simulink model "Microgrid_PV_WG_Bat_EV_j_22b"  (R2022b)
settings: Solver=VariableStepAuto  StartTime=0.0  StopTime=1  RelTol=1e-3
undefined symbols (not defined in the file or in its folder): Acid, Ion, Lead, Lithium
libraries: slpidlib x35, spsabctodq0Lib x23, spsSeriesRLCBranchLib x19, spsCurrentMeasurementLib x13, spsVoltageMeasurementLib x11, spsThreePhaseVIMeasurementLib x10, spsPLL3phLib x9, spsThreePhaseSeriesRLCBranchLib x9, spsPower3phInstantaneousLib x8, spsIGBTDiodeLib x8, spsUniversalBridgeLib x7, spsPWMGeneratorDCDCLib x6
(part 2 of 5)

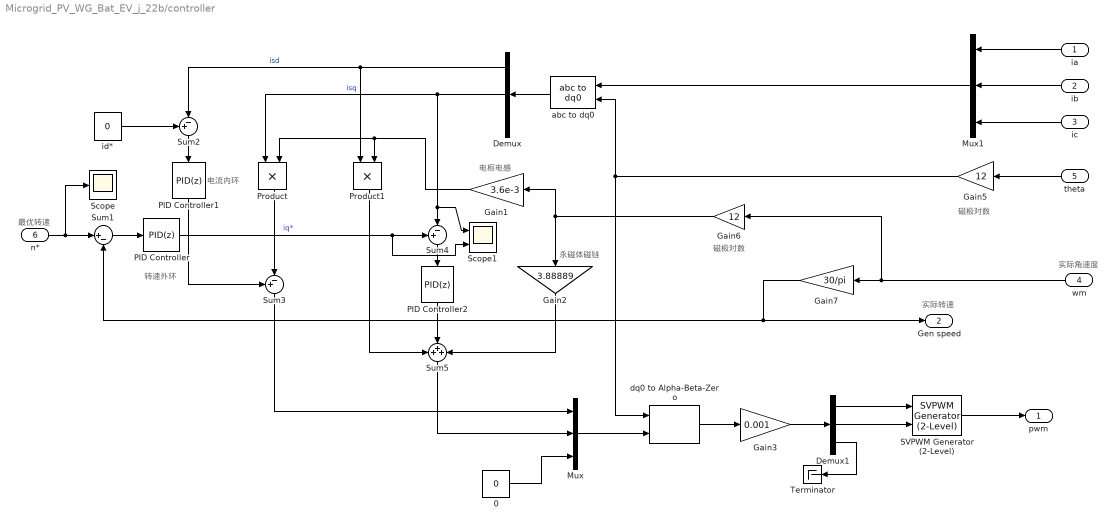
== system Microgrid_PV_WG_Bat_EV_j_22b/controller ==
  note: 电枢电感
  note: 永磁体磁链
  note: 实际角速度
  note: 实际转速
  note: 最优转速
  note: 电流内环
  note: 转速外环
  note: 磁极对数
  note: 磁极对数
  ia : Inport
  ib : Inport  Port=2
  ic : Inport  Port=3
  wm : Inport  Port=4
  theta : Inport  Port=5
  n* : Inport  Port=6
  0 : Constant  Value=0
  Demux : Demux  Outputs=3
  Demux1 : Demux  Outputs=3
  Gain1 : Gain  Gain=3.6e-3
  Gain2 : Gain  Gain=3.88889
  Gain3 : Gain  Gain=0.001
  Gain5 : Gain  Gain=12
  Gain6 : Gain  Gain=12
  Gain7 : Gain  Gain=30/pi
  Mux : Mux  Inputs=3
  Mux1 : Mux  Inputs=3
  PID Controller : slpidlib/PID Controller  Controller=PID  Form=Parallel  TimeDomain=Discrete-time  UseExternalTs=off  SampleTime=1e-5  IntegratorMethod=Forward Euler  FilterMethod=Forward Euler  ControllerParametersSource=internal  P=20  I=400  UseKiTs=off  D=0  N=100  UseFilter=on  TunerSelectOption=Transfer Function Based (PID Tuner App)  InitialConditionSource=internal  InitialConditionForIntegrator=0  InitialConditionForFilter=0  DifferentiatorICPrevScaledInput=0  ExternalReset=none  TrackingMode=off  Kt=1  LimitOutput=off  SatLimitsSource=internal  UpperSaturationLimit=inf  LowerSaturationLimit=-inf  LinearizeAsGain=on  AntiWindupMode=none  Kb=1  LimitIntegrator=off  UpperIntegratorSaturationLimit=inf  LowerIntegratorSaturationLimit=-inf  POutMin=[]  POutMax=[]  IOutMin=[]  IOutMax=[]  DOutMin=[]  DOutMax=[]  NOutMin=[]  NOutMax=[]  SumOutMin=[]  SumOutMax=[]  SaturationOutMin=[]  SaturationOutMax=[]  PParamMin=[]  PParamMax=[]  IParamMin=[]  IParamMax=[]  DParamMin=[]  DParamMax=[]  NParamMin=[]  NParamMax=[]  KbParamMin=[]  KbParamMax=[]  KtParamMin=[]  KtParamMax=[]  KbOutMin=[]  KbOutMax=[]  KtOutMin=[]  KtOutMax=[]  IntegratorOutMin=[]  IntegratorOutMax=[]  FilterOutMin=[]  FilterOutMax=[]  SumI1OutMin=[]  SumI1OutMax=[]  SumI2OutMin=[]  SumI2OutMax=[]  SumI3OutMin=[]  SumI3OutMax=[]  SumI4OutMin=[]  SumI4OutMax=[]  SumDOutMin=[]  SumDOutMax=[]  DifferentiatorOutMin=[]  DifferentiatorOutMax=[]  FilterDiffOutCoefMin=[]  FilterDiffOutCoefMax=[]  ReciprocalOutMin=[]  ReciprocalOutMax=[]  SumDenOutMin=[]  SumDenOutMax=[]  SumNumOutMin=[]  SumNumOutMax=[]  DivideOutMin=[]  DivideOutMax=[]  UdiffTsProdOutMin=[]  UdiffTsProdOutMax=[]  NTsProdOutMin=[]  NTsProdOutMax=[]  UintegralTsProdOutMin=[]  UintegralTsProdOutMax=[]  UngainTsProdOutMin=[]  UngainTsProdOutMax=[]  IntegratorContinuousStateAttributes=''  IntegratorStateMustResolveToSignalObject=off  IntegratorRTWStateStorageClass=Auto  FilterContinuousStateAttributes=''  FilterStateMustResolveToSignalObject=off  FilterRTWStateStorageClass=Auto  ParallelPVariant=InternalParameters  IdealPVariant=Disabled  IVariant=InternalParameters  DVariant=InternalParameters  IntegratorVariant=Discrete  SatVariant=Disabled  AWVariant=Passthrough  PCopyVariant=Disabled  TRVariant=Disabled  FdbkBlocksVariant=Forward  IdealPFdbkVariant=Disabled  SatFdbkVariant=Disabled  DerivativeFilterVariant=ForwardEulerFilter  NVariant=InternalParameters  NCopyVariant=Disabled  FilterICVariant=InternalICsFilter  IntegratorICVariant=InternalICs  ExternalResetVariant=Disabled  TRSumVariant=Passthrough  SumFdbkVariant=Disabled  SumVariant=Sum_PID  TsampFilterVariant=InternalTs  TsampNgainVariant=Passthrough  TsampIntegralVariant=Disabled_SignalSpec  ExternalSaturationOutDataTypeStr=Inherit: Same as second input
  PID Controller1 : slpidlib/PID Controller  Controller=PID  Form=Parallel  TimeDomain=Discrete-time  UseExternalTs=off  SampleTime=1e-5  IntegratorMethod=Forward Euler  FilterMethod=Forward Euler  ControllerParametersSource=internal  P=5  I=100  UseKiTs=off  D=0  N=100  UseFilter=on  TunerSelectOption=Transfer Function Based (PID Tuner App)  InitialConditionSource=internal  InitialConditionForIntegrator=0  InitialConditionForFilter=0  DifferentiatorICPrevScaledInput=0  ExternalReset=none  TrackingMode=off  Kt=1  LimitOutput=off  SatLimitsSource=internal  UpperSaturationLimit=inf  LowerSaturationLimit=-inf  LinearizeAsGain=on  AntiWindupMode=none  Kb=1  LimitIntegrator=off  UpperIntegratorSaturationLimit=inf  LowerIntegratorSaturationLimit=-inf  POutMin=[]  POutMax=[]  IOutMin=[]  IOutMax=[]  DOutMin=[]  DOutMax=[]  NOutMin=[]  NOutMax=[]  SumOutMin=[]  SumOutMax=[]  SaturationOutMin=[]  SaturationOutMax=[]  PParamMin=[]  PParamMax=[]  IParamMin=[]  IParamMax=[]  DParamMin=[]  DParamMax=[]  NParamMin=[]  NParamMax=[]  KbParamMin=[]  KbParamMax=[]  KtParamMin=[]  KtParamMax=[]  KbOutMin=[]  KbOutMax=[]  KtOutMin=[]  KtOutMax=[]  IntegratorOutMin=[]  IntegratorOutMax=[]  FilterOutMin=[]  FilterOutMax=[]  SumI1OutMin=[]  SumI1OutMax=[]  SumI2OutMin=[]  SumI2OutMax=[]  SumI3OutMin=[]  SumI3OutMax=[]  SumI4OutMin=[]  SumI4OutMax=[]  SumDOutMin=[]  SumDOutMax=[]  DifferentiatorOutMin=[]  DifferentiatorOutMax=[]  FilterDiffOutCoefMin=[]  FilterDiffOutCoefMax=[]  ReciprocalOutMin=[]  ReciprocalOutMax=[]  SumDenOutMin=[]  SumDenOutMax=[]  SumNumOutMin=[]  SumNumOutMax=[]  DivideOutMin=[]  DivideOutMax=[]  UdiffTsProdOutMin=[]  UdiffTsProdOutMax=[]  NTsProdOutMin=[]  NTsProdOutMax=[]  UintegralTsProdOutMin=[]  UintegralTsProdOutMax=[]  UngainTsProdOutMin=[]  UngainTsProdOutMax=[]  IntegratorContinuousStateAttributes=''  IntegratorStateMustResolveToSignalObject=off  IntegratorRTWStateStorageClass=Auto  FilterContinuousStateAttributes=''  FilterStateMustResolveToSignalObject=off  FilterRTWStateStorageClass=Auto  ParallelPVariant=InternalParameters  IdealPVariant=Disabled  IVariant=InternalParameters  DVariant=InternalParameters  IntegratorVariant=Discrete  SatVariant=Disabled  AWVariant=Passthrough  PCopyVariant=Disabled  TRVariant=Disabled  FdbkBlocksVariant=Forward  IdealPFdbkVariant=Disabled  SatFdbkVariant=Disabled  DerivativeFilterVariant=ForwardEulerFilter  NVariant=InternalParameters  NCopyVariant=Disabled  FilterICVariant=InternalICsFilter  IntegratorICVariant=InternalICs  ExternalResetVariant=Disabled  TRSumVariant=Passthrough  SumFdbkVariant=Disabled  SumVariant=Sum_PID  TsampFilterVariant=InternalTs  TsampNgainVariant=Passthrough  TsampIntegralVariant=Disabled_SignalSpec  ExternalSaturationOutDataTypeStr=Inherit: Same as second input
  PID Controller2 : slpidlib/PID Controller  Controller=PID  Form=Parallel  TimeDomain=Discrete-time  UseExternalTs=off  SampleTime=1e-5  IntegratorMethod=Forward Euler  FilterMethod=Forward Euler  ControllerParametersSource=internal  P=5  I=100  UseKiTs=off  D=0  N=100  UseFilter=on  TunerSelectOption=Transfer Function Based (PID Tuner App)  InitialConditionSource=internal  InitialConditionForIntegrator=0  InitialConditionForFilter=0  DifferentiatorICPrevScaledInput=0  ExternalReset=none  TrackingMode=off  Kt=1  LimitOutput=off  SatLimitsSource=internal  UpperSaturationLimit=inf  LowerSaturationLimit=-inf  LinearizeAsGain=on  AntiWindupMode=none  Kb=1  LimitIntegrator=off  UpperIntegratorSaturationLimit=inf  LowerIntegratorSaturationLimit=-inf  POutMin=[]  POutMax=[]  IOutMin=[]  IOutMax=[]  DOutMin=[]  DOutMax=[]  NOutMin=[]  NOutMax=[]  SumOutMin=[]  SumOutMax=[]  SaturationOutMin=[]  SaturationOutMax=[]  PParamMin=[]  PParamMax=[]  IParamMin=[]  IParamMax=[]  DParamMin=[]  DParamMax=[]  NParamMin=[]  NParamMax=[]  KbParamMin=[]  KbParamMax=[]  KtParamMin=[]  KtParamMax=[]  KbOutMin=[]  KbOutMax=[]  KtOutMin=[]  KtOutMax=[]  IntegratorOutMin=[]  IntegratorOutMax=[]  FilterOutMin=[]  FilterOutMax=[]  SumI1OutMin=[]  SumI1OutMax=[]  SumI2OutMin=[]  SumI2OutMax=[]  SumI3OutMin=[]  SumI3OutMax=[]  SumI4OutMin=[]  SumI4OutMax=[]  SumDOutMin=[]  SumDOutMax=[]  DifferentiatorOutMin=[]  DifferentiatorOutMax=[]  FilterDiffOutCoefMin=[]  FilterDiffOutCoefMax=[]  ReciprocalOutMin=[]  ReciprocalOutMax=[]  SumDenOutMin=[]  SumDenOutMax=[]  SumNumOutMin=[]  SumNumOutMax=[]  DivideOutMin=[]  DivideOutMax=[]  UdiffTsProdOutMin=[]  UdiffTsProdOutMax=[]  NTsProdOutMin=[]  NTsProdOutMax=[]  UintegralTsProdOutMin=[]  UintegralTsProdOutMax=[]  UngainTsProdOutMin=[]  UngainTsProdOutMax=[]  IntegratorContinuousStateAttributes=''  IntegratorStateMustResolveToSignalObject=off  IntegratorRTWStateStorageClass=Auto  FilterContinuousStateAttributes=''  FilterStateMustResolveToSignalObject=off  FilterRTWStateStorageClass=Auto  ParallelPVariant=InternalParameters  IdealPVariant=Disabled  IVariant=InternalParameters  DVariant=InternalParameters  IntegratorVariant=Discrete  SatVariant=Disabled  AWVariant=Passthrough  PCopyVariant=Disabled  TRVariant=Disabled  FdbkBlocksVariant=Forward  IdealPFdbkVariant=Disabled  SatFdbkVariant=Disabled  DerivativeFilterVariant=ForwardEulerFilter  NVariant=InternalParameters  NCopyVariant=Disabled  FilterICVariant=InternalICsFilter  IntegratorICVariant=InternalICs  ExternalResetVariant=Disabled  TRSumVariant=Passthrough  SumFdbkVariant=Disabled  SumVariant=Sum_PID  TsampFilterVariant=InternalTs  TsampNgainVariant=Passthrough  TsampIntegralVariant=Disabled_SignalSpec  ExternalSaturationOutDataTypeStr=Inherit: Same as second input
  Product : Product
  Product1 : Product
  SVPWM Generator (2-Level) : spsSVPWMGenerator2LevelLib/SVPWM Generator (2-Level)  InputType=alpha-beta components  SwitchingPattern=Pattern #1  Fc=3000  ParUref=[0.8 -30 50]  Ts=0
  Scope : Scope
  Scope1 : Scope  NumInputPorts=2
  Sum1 : Sum  Inputs=|+-
  Sum2 : Sum  Inputs=+-|
  Sum3 : Sum  Inputs=+-|
  Sum4 : Sum  Inputs=+-|
  Sum5 : Sum  Inputs=+++
  Terminator : Terminator
  abc to dq0 : spsabctodq0Lib/abc to dq0  Alignment=90 degrees behind phase A axis
  dq0 to Alpha-Beta-Zero : spsdq0toAlphaBetaZeroLib/dq0 to Alpha-Beta-Zero  Alignment=90 degrees behind phase A axis
  id* : Constant  Value=0
  pwm : Outport
  Gen speed : Outport  Port=2
  wires:
  Demux1/1 -> SVPWM Generator (2-Level)/1
  Gain5/1 -> dq0 to Alpha-Beta-Zero/2, abc to dq0/2
  Gain7/1 -> Gen speed/1, Sum1/2
  Mux/1 -> dq0 to Alpha-Beta-Zero/1
  wm/1 -> Gain6/1, Gain7/1
  Mux1/1 -> abc to dq0/1
  ib/1 -> Mux1/2
  Sum3/1 -> Mux/1
  PID Controller2/1 -> Sum5/2
  Sum1/1 -> PID Controller/1
  0/1 -> Mux/3
  Gain6/1 -> Gain1/1, Gain2/1
  theta/1 -> Gain5/1
  Demux/2 -> Scope1/1, Sum4/2, Product/1  "isq"
  Demux1/3 -> Terminator/1
  Gain3/1 -> Demux1/1
  dq0 to Alpha-Beta-Zero/1 -> Gain3/1
  Sum5/1 -> Mux/2
  Demux/1 -> Sum2/2, Product1/1  "isd"
  id*/1 -> Sum2/1
  Gain1/1 -> Product1/2, Product/2
  ia/1 -> Mux1/1
  PID Controller1/1 -> Sum3/1
  SVPWM Generator (2-Level)/1 -> pwm/1
  Product1/1 -> Sum5/1
  Demux1/2 -> SVPWM Generator (2-Level)/2
  Product/1 -> Sum3/2
  PID Controller/1 -> Scope1/2, Sum4/1  "iq*"
  Sum2/1 -> PID Controller1/1
  Gain2/1 -> Sum5/3
  Sum4/1 -> PID Controller2/1
  ic/1 -> Mux1/3
  abc to dq0/1 -> Demux/1
  n*/1 -> Scope/1, Sum1/1

== system Microgrid_PV_WG_Bat_EV_j_22b/controller2 ==
  note: abc2dq
  Udc : Inport
  Udc_ref : Inport  Port=2
  Vabc : Inport  Port=3
  Iabc : Inport  Port=4
  Constant : Constant  Commented=on  Value=600
  Constant4 : Constant  Value=0
  Demux2 : Demux  Outputs=3
  Demux3 : Demux  Outputs=3
  Demux4 : Demux  Outputs=3
  Gain6 : Gain  Gain=2*pi*50*(7e-3)
  Gain7 : Gain  Gain=2*pi*50*(7e-3)
  Gain9 : Gain  Gain=0.001
  Mux1 : Mux  Inputs=3
  PID 3 : slpidlib/PID Controller  Controller=PID  Form=Parallel  TimeDomain=Discrete-time  UseExternalTs=off  SampleTime=1e-5  IntegratorMethod=Forward Euler  FilterMethod=Forward Euler  ControllerParametersSource=internal  P=2  I=70  UseKiTs=off  D=0  N=100  UseFilter=on  TunerSelectOption=Transfer Function Based (PID Tuner App)  InitialConditionSource=internal  InitialConditionForIntegrator=0  InitialConditionForFilter=0  DifferentiatorICPrevScaledInput=0  ExternalReset=none  TrackingMode=off  Kt=1  LimitOutput=off  SatLimitsSource=internal  UpperSaturationLimit=inf  LowerSaturationLimit=-inf  LinearizeAsGain=on  AntiWindupMode=none  Kb=1  LimitIntegrator=off  UpperIntegratorSaturationLimit=inf  LowerIntegratorSaturationLimit=-inf  POutMin=[]  POutMax=[]  IOutMin=[]  IOutMax=[]  DOutMin=[]  DOutMax=[]  NOutMin=[]  NOutMax=[]  SumOutMin=[]  SumOutMax=[]  SaturationOutMin=[]  SaturationOutMax=[]  PParamMin=[]  PParamMax=[]  IParamMin=[]  IParamMax=[]  DParamMin=[]  DParamMax=[]  NParamMin=[]  NParamMax=[]  KbParamMin=[]  KbParamMax=[]  KtParamMin=[]  KtParamMax=[]  KbOutMin=[]  KbOutMax=[]  KtOutMin=[]  KtOutMax=[]  IntegratorOutMin=[]  IntegratorOutMax=[]  FilterOutMin=[]  FilterOutMax=[]  SumI1OutMin=[]  SumI1OutMax=[]  SumI2OutMin=[]  SumI2OutMax=[]  SumI3OutMin=[]  SumI3OutMax=[]  SumI4OutMin=[]  SumI4OutMax=[]  SumDOutMin=[]  SumDOutMax=[]  DifferentiatorOutMin=[]  DifferentiatorOutMax=[]  FilterDiffOutCoefMin=[]  FilterDiffOutCoefMax=[]  ReciprocalOutMin=[]  ReciprocalOutMax=[]  SumDenOutMin=[]  SumDenOutMax=[]  SumNumOutMin=[]  SumNumOutMax=[]  DivideOutMin=[]  DivideOutMax=[]  UdiffTsProdOutMin=[]  UdiffTsProdOutMax=[]  NTsProdOutMin=[]  NTsProdOutMax=[]  UintegralTsProdOutMin=[]  UintegralTsProdOutMax=[]  UngainTsProdOutMin=[]  UngainTsProdOutMax=[]  IntegratorContinuousStateAttributes=''  IntegratorStateMustResolveToSignalObject=off  IntegratorRTWStateStorageClass=Auto  FilterContinuousStateAttributes=''  FilterStateMustResolveToSignalObject=off  FilterRTWStateStorageClass=Auto  ParallelPVariant=InternalParameters  IdealPVariant=Disabled  IVariant=InternalParameters  DVariant=InternalParameters  IntegratorVariant=Discrete  SatVariant=Disabled  AWVariant=Passthrough  PCopyVariant=Disabled  TRVariant=Disabled  FdbkBlocksVariant=Forward  IdealPFdbkVariant=Disabled  SatFdbkVariant=Disabled  DerivativeFilterVariant=ForwardEulerFilter  NVariant=InternalParameters  NCopyVariant=Disabled  FilterICVariant=InternalICsFilter  IntegratorICVariant=InternalICs  ExternalResetVariant=Disabled  TRSumVariant=Passthrough  SumFdbkVariant=Disabled  SumVariant=Sum_PID  TsampFilterVariant=InternalTs  TsampNgainVariant=Passthrough  TsampIntegralVariant=Disabled_SignalSpec  ExternalSaturationOutDataTypeStr=Inherit: Same as second input
  PID 4 : slpidlib/PID Controller  Controller=PID  Form=Parallel  TimeDomain=Discrete-time  UseExternalTs=off  SampleTime=1e-5  IntegratorMethod=Forward Euler  FilterMethod=Forward Euler  ControllerParametersSource=internal  P=1  I=15  UseKiTs=off  D=0  N=100  UseFilter=on  TunerSelectOption=Transfer Function Based (PID Tuner App)  InitialConditionSource=internal  InitialConditionForIntegrator=0  InitialConditionForFilter=0  DifferentiatorICPrevScaledInput=0  ExternalReset=none  TrackingMode=off  Kt=1  LimitOutput=off  SatLimitsSource=internal  UpperSaturationLimit=inf  LowerSaturationLimit=-inf  LinearizeAsGain=on  AntiWindupMode=none  Kb=1  LimitIntegrator=off  UpperIntegratorSaturationLimit=inf  LowerIntegratorSaturationLimit=-inf  POutMin=[]  POutMax=[]  IOutMin=[]  IOutMax=[]  DOutMin=[]  DOutMax=[]  NOutMin=[]  NOutMax=[]  SumOutMin=[]  SumOutMax=[]  SaturationOutMin=[]  SaturationOutMax=[]  PParamMin=[]  PParamMax=[]  IParamMin=[]  IParamMax=[]  DParamMin=[]  DParamMax=[]  NParamMin=[]  NParamMax=[]  KbParamMin=[]  KbParamMax=[]  KtParamMin=[]  KtParamMax=[]  KbOutMin=[]  KbOutMax=[]  KtOutMin=[]  KtOutMax=[]  IntegratorOutMin=[]  IntegratorOutMax=[]  FilterOutMin=[]  FilterOutMax=[]  SumI1OutMin=[]  SumI1OutMax=[]  SumI2OutMin=[]  SumI2OutMax=[]  SumI3OutMin=[]  SumI3OutMax=[]  SumI4OutMin=[]  SumI4OutMax=[]  SumDOutMin=[]  SumDOutMax=[]  DifferentiatorOutMin=[]  DifferentiatorOutMax=[]  FilterDiffOutCoefMin=[]  FilterDiffOutCoefMax=[]  ReciprocalOutMin=[]  ReciprocalOutMax=[]  SumDenOutMin=[]  SumDenOutMax=[]  SumNumOutMin=[]  SumNumOutMax=[]  DivideOutMin=[]  DivideOutMax=[]  UdiffTsProdOutMin=[]  UdiffTsProdOutMax=[]  NTsProdOutMin=[]  NTsProdOutMax=[]  UintegralTsProdOutMin=[]  UintegralTsProdOutMax=[]  UngainTsProdOutMin=[]  UngainTsProdOutMax=[]  IntegratorContinuousStateAttributes=''  IntegratorStateMustResolveToSignalObject=off  IntegratorRTWStateStorageClass=Auto  FilterContinuousStateAttributes=''  FilterStateMustResolveToSignalObject=off  FilterRTWStateStorageClass=Auto  ParallelPVariant=InternalParameters  IdealPVariant=Disabled  IVariant=InternalParameters  DVariant=InternalParameters  IntegratorVariant=Discrete  SatVariant=Disabled  AWVariant=Passthrough  PCopyVariant=Disabled  TRVariant=Disabled  FdbkBlocksVariant=Forward  IdealPFdbkVariant=Disabled  SatFdbkVariant=Disabled  DerivativeFilterVariant=ForwardEulerFilter  NVariant=InternalParameters  NCopyVariant=Disabled  FilterICVariant=InternalICsFilter  IntegratorICVariant=InternalICs  ExternalResetVariant=Disabled  TRSumVariant=Passthrough  SumFdbkVariant=Disabled  SumVariant=Sum_PID  TsampFilterVariant=InternalTs  TsampNgainVariant=Passthrough  TsampIntegralVariant=Disabled_SignalSpec  ExternalSaturationOutDataTypeStr=Inherit: Same as second input
  PID 5 : slpidlib/PID Controller  Controller=PID  Form=Parallel  TimeDomain=Discrete-time  UseExternalTs=off  SampleTime=1e-5  IntegratorMethod=Forward Euler  FilterMethod=Forward Euler  ControllerParametersSource=internal  P=1  I=15  UseKiTs=off  D=0  N=100  UseFilter=on  TunerSelectOption=Transfer Function Based (PID Tuner App)  InitialConditionSource=internal  InitialConditionForIntegrator=0  InitialConditionForFilter=0  DifferentiatorICPrevScaledInput=0  ExternalReset=none  TrackingMode=off  Kt=1  LimitOutput=off  SatLimitsSource=internal  UpperSaturationLimit=inf  LowerSaturationLimit=-inf  LinearizeAsGain=on  AntiWindupMode=none  Kb=1  LimitIntegrator=off  UpperIntegratorSaturationLimit=inf  LowerIntegratorSaturationLimit=-inf  POutMin=[]  POutMax=[]  IOutMin=[]  IOutMax=[]  DOutMin=[]  DOutMax=[]  NOutMin=[]  NOutMax=[]  SumOutMin=[]  SumOutMax=[]  SaturationOutMin=[]  SaturationOutMax=[]  PParamMin=[]  PParamMax=[]  IParamMin=[]  IParamMax=[]  DParamMin=[]  DParamMax=[]  NParamMin=[]  NParamMax=[]  KbParamMin=[]  KbParamMax=[]  KtParamMin=[]  KtParamMax=[]  KbOutMin=[]  KbOutMax=[]  KtOutMin=[]  KtOutMax=[]  IntegratorOutMin=[]  IntegratorOutMax=[]  FilterOutMin=[]  FilterOutMax=[]  SumI1OutMin=[]  SumI1OutMax=[]  SumI2OutMin=[]  SumI2OutMax=[]  SumI3OutMin=[]  SumI3OutMax=[]  SumI4OutMin=[]  SumI4OutMax=[]  SumDOutMin=[]  SumDOutMax=[]  DifferentiatorOutMin=[]  DifferentiatorOutMax=[]  FilterDiffOutCoefMin=[]  FilterDiffOutCoefMax=[]  ReciprocalOutMin=[]  ReciprocalOutMax=[]  SumDenOutMin=[]  SumDenOutMax=[]  SumNumOutMin=[]  SumNumOutMax=[]  DivideOutMin=[]  DivideOutMax=[]  UdiffTsProdOutMin=[]  UdiffTsProdOutMax=[]  NTsProdOutMin=[]  NTsProdOutMax=[]  UintegralTsProdOutMin=[]  UintegralTsProdOutMax=[]  UngainTsProdOutMin=[]  UngainTsProdOutMax=[]  IntegratorContinuousStateAttributes=''  IntegratorStateMustResolveToSignalObject=off  IntegratorRTWStateStorageClass=Auto  FilterContinuousStateAttributes=''  FilterStateMustResolveToSignalObject=off  FilterRTWStateStorageClass=Auto  ParallelPVariant=InternalParameters  IdealPVariant=Disabled  IVariant=InternalParameters  DVariant=InternalParameters  IntegratorVariant=Discrete  SatVariant=Disabled  AWVariant=Passthrough  PCopyVariant=Disabled  TRVariant=Disabled  FdbkBlocksVariant=Forward  IdealPFdbkVariant=Disabled  SatFdbkVariant=Disabled  DerivativeFilterVariant=ForwardEulerFilter  NVariant=InternalParameters  NCopyVariant=Disabled  FilterICVariant=InternalICsFilter  IntegratorICVariant=InternalICs  ExternalResetVariant=Disabled  TRSumVariant=Passthrough  SumFdbkVariant=Disabled  SumVariant=Sum_PID  TsampFilterVariant=InternalTs  TsampNgainVariant=Passthrough  TsampIntegralVariant=Disabled_SignalSpec  ExternalSaturationOutDataTypeStr=Inherit: Same as second input
  PLL (3ph)1 : spsPLL3phLib/PLL (3ph)  Fmin=45  Par_Init=[0, 50]  ParK=[180, 3200, 1]  TcD=1e-4  MaxRateChangeFreq=12  FilterCutOffFreq=25  Ts=0  AGC=on
  SVPWM Generator (2-Level)1 : spsSVPWMGenerator2LevelLib/SVPWM Generator (2-Level)  InputType=alpha-beta components  SwitchingPattern=Pattern #1  Fc=10000  ParUref=[0.8 -30 50]  Ts=0
  Sum1 : Sum  Commented=on  Inputs=|+-
  Sum5 : Sum  Inputs=|+-
  Sum6 : Sum  Inputs=|+-
  Sum7 : Sum  Inputs=++-
  Sum8 : Sum  Inputs=-+|
  Sum9 : Sum  Inputs=+++
  Terminator2 : Terminator
  Terminator3 : Terminator
  Terminator4 : Terminator
  abc to dq1 : spsabctodq0Lib/abc to dq0  Alignment=90 degrees behind phase A axis
  abc to dq2 : spsabctodq0Lib/abc to dq0  Alignment=90 degrees behind phase A axis
  dq0 to Alpha-Beta-Zero1 : spsdq0toAlphaBetaZeroLib/dq0 to Alpha-Beta-Zero  Alignment=90 degrees behind phase A axis
  iq*=0 : Constant  Value=0
  Pulse : Outport
  wires:
  Sum5/1 -> PID 3/1  "d"
  Gain6/1 -> Sum7/3
  Demux2/1 -> Sum7/1  "Vd"
  PID 3/1 -> Sum6/1  "id*"
  dq0 to Alpha-Beta-Zero1/1 -> Gain9/1
  PLL (3ph)1/2 -> dq0 to Alpha-Beta-Zero1/2, abc to dq2/2, abc to dq1/2
  Sum6/1 -> PID 4/1
  PID 4/1 -> Sum7/2
  Demux4/3 -> Terminator4/1
  PID 5/1 -> Sum9/2
  Iabc/1 -> abc to dq2/1
  Constant4/1 -> Mux1/3
  Demux3/3 -> Terminator3/1
  abc to dq1/1 -> Demux2/1
  Demux2/3 -> Terminator2/1
  Udc/1 -> Sum5/1
  abc to dq2/1 -> Demux3/1
  iq*=0/1 -> Sum8/2
  SVPWM Generator (2-Level)1/1 -> Pulse/1
  Gain9/1 -> Demux4/1
  Demux3/2 -> Sum8/1, Gain6/1  "iq"
  Demux3/1 -> Gain7/1, Sum6/2  "id"
  Sum7/1 -> Mux1/1  "Ud*"
  Sum8/1 -> PID 5/1
  Sum9/1 -> Mux1/2  "Uq*"
  Mux1/1 -> dq0 to Alpha-Beta-Zero1/1
  Demux4/1 -> SVPWM Generator (2-Level)1/1
  Demux4/2 -> SVPWM Generator (2-Level)1/2
  Udc_ref/1 -> Sum5/2
  Gain7/1 -> Sum9/3
  Demux2/2 -> Sum9/1  "Vq"
  Vabc/1 -> PLL (3ph)1/1, abc to dq1/1  "d"
  Constant/1 -> Sum1/2

== system Microgrid_PV_WG_Bat_EV_j_22b/储氢罐 ==
  Velec : Inport
  L/min : Inport  Port=2
  Add1 : Sum  Inputs=+-
  Add2 : Sum
  Add3 : Sum
  Divide1 : Product  Inputs=*/
  Gain : Gain  Gain=10
  Gain1 : Gain  Gain=30
  Integrator : Integrator
  Product1 : Product  Inputs=***/
  R : Constant  Value=8.3145
  T/C : Constant  Value=25
  conversion : Constant  Value=273.15
  储氢罐的体积/m³ : Constant
  标准大气压/pa : Constant  Value=101325
  标准大气压/pa1 : Constant  Value=101325
  氢气消耗速率转换 : Subsystem
  百分比 : Gain  Gain=100
  SOH : Outport
  wires:
  R/1 -> Product1/2
  Gain/1 -> Add3/2  "储氢罐已有氢气的压强"
  Integrator/1 -> Product1/1
  T/C/1 -> Add2/1
  conversion/1 -> Add2/2
  标准大气压/pa/1 -> Gain/1
  Velec/1 -> Add1/1
  标准大气压/pa1/1 -> Gain1/1
  储氢罐的体积/m³/1 -> Product1/4
  氢气消耗速率转换/1(mol/s) -> Add1/2
  Divide1/1 -> 百分比/1
  Add3/1 -> Divide1/1
  Product1/1 -> Add3/1
  百分比/1 -> SOH/1
  Gain1/1 -> Divide1/2  "储氢罐最大储氢的氢气的压强"
  Add2/1 -> Product1/3  "T/K"
  Add1/1 -> Integrator/1
  L/min/1 -> 氢气消耗速率转换/1(L/min)

== system Microgrid_PV_WG_Bat_EV_j_22b/充电桩 ==
  Battery1 : spsBatteryLib/Battery  BatType=Lead-Acid  ShowTempParam=off  ThermalPreset=no  ShowAgeParam=off  NomV=500  NomQ=1000  SOC=50  Batt_Tr=30  PresetModel=on  MaxQ=1041.6667  MinV=375  FullV=544.4079  Dis_rate=200  R=0.005  Normal_OP=310.2778  expZone="[509.0461      3.333333]"  current=[6.5 13 32.5]  Units=Time  Tci=20  NomT=20  T2=-30  MaxQ2=4.8  FullV2=7.1  Normal_OP2=5.655  expZone2="[6.58           1]"  Rca=0.6  ti=2000  Dp=0  Neq0=0  Tsim=1e6  Ta1=25  Qeol=5.4*0.9  Reol=0.013333*1.2  Char_age=[2.3478, 3]  Dis_age=[2.3478, 10]  N1=1500  N2=10500  N3=1000  N4=1400  Ta2=45  N5=950
  Bus Selector1 : BusSelector  OutputSignals=SOC (%),Current (A),Voltage (V)
  Current Measurement2 : spsCurrentMeasurementLib/Current Measurement  PhasorSimulation=off  OutputType=Complex  PSBequivalent=0
  IGBT/Diode2 : spsIGBTDiodeLib/IGBT//Diode  Ron=1e-3  Rs=1e5  Cs=inf  Measurements=on
  IGBT/Diode3 : spsIGBTDiodeLib/IGBT//Diode  Ron=1e-3  Rs=1e5  Cs=inf  Measurements=on
  Mosfet : spsMosfetLib/Mosfet  Ron=0.1  Lon=0  Rd=0.01  Vfd=0  IC=0  Rs=1e5  Cs=inf  Measurements=on
  PWM Generator (DC-DC)2 : spsPWMGeneratorDCDCLib/PWM Generator (DC-DC)  Fsw=1e4  Ts=0
  Scope : Scope
  Scope3 : Scope  NumInputPorts=2
  Scope5 : Scope  NumInputPorts=3
  Series RLC Branch3 : spsSeriesRLCBranchLib/Series RLC Branch  LConnTagsString=__new0  RConnTagsString=__new0  BranchType=L  Resistance=1  Inductance=11e-2  SetiL0=off  InitialCurrent=0  Capacitance=1e-6  Setx0=off  InitialVoltage=0  Measurements=None
  Series RLC Branch5 : spsSeriesRLCBranchLib/Series RLC Branch  LConnTagsString=__new0  RConnTagsString=__new0  BranchType=RC  Resistance=0.01  Inductance=1e-3  SetiL0=off  InitialCurrent=0  Capacitance=2e-2  Setx0=off  InitialVoltage=10  Measurements=None
  Voltage Measurement1 : spsVoltageMeasurementLib/Voltage Measurement  PhasorSimulation=off  OutputType=Complex  PSBequivalent=0
  恒流恒压充电 : Subsystem
  + : PMIOPort  Side=Right
  - : PMIOPort  Port=2  Side=Right
  Vbat : Outport
  Ibat : Outport  Port=2
  SOC : Outport  Port=3
  wires:
  恒流恒压充电/1(D) -> PWM Generator (DC-DC)2/1, Scope/1
  Bus Selector1/2 -> Scope5/2, [I_Bat]  "<Current (A)>"
  Bus Selector1/1 -> Scope5/1, [SOC]  "<SOC (%)>"
  Voltage Measurement1/1 -> 恒流恒压充电/1(V), Scope3/2
  PWM Generator (DC-DC)2/1 -> Mosfet/1
  Current Measurement2/1 -> Scope3/1, 恒流恒压充电/2(I)
  Battery1/1 -> Bus Selector1/1
  [I_Bat] -> Ibat/1
  Bus Selector1/3 -> Scope5/3, [V_Bat]  "<Voltage (V)>"
  [V_Bat] -> Vbat/1
  [SOC] -> SOC/1
  connections:
  IGBT/Diode2/RConn1 -- Voltage Measurement1/LConn2 -- Battery1/LConn2 -- Series RLC Branch5/RConn1 -- -/RConn1
  Current Measurement2/LConn1 -- Series RLC Branch5/LConn1 -- Series RLC Branch3/RConn1
  +/RConn1 -- Mosfet/LConn1
  IGBT/Diode3/RConn1 -- Current Measurement2/RConn1
  Voltage Measurement1/LConn1 -- IGBT/Diode3/LConn1 -- Battery1/LConn1
  Mosfet/RConn1 -- IGBT/Diode2/LConn1 -- Series RLC Branch3/LConn1

== system Microgrid_PV_WG_Bat_EV_j_22b/光伏 ==
  PV_change : Inport
  Bus Selector : BusSelector  OutputSignals=V_PV,I_PV
  Constant : Constant  Value=25
  Constant1 : Constant  Value=1000
  Constant2 : Constant  Value=1000
  Current Measurement : spsCurrentMeasurementLib/Current Measurement  PhasorSimulation=off  OutputType=Complex  PSBequivalent=0
  Diode : spsDiodeLib/Diode  Ron=0.001  Lon=0  Vf=0.8  IC=0  UseSnubber=0  Rs=500  Cs=250e-9  Measurements=on
  IGBT : spsIGBTLib/IGBT  Ron=0.001  Lon=0  Vf=1  Tf=1e-6  Tt=2e-6  IC=0  Rs=1e5  Cs=inf  Measurements=on
  "PV Array " : spsPVArrayLib/PV Array  Npar=5  Nser=14  PlotType=array @ 25 deg.C & specified irradiances  S_vec="[ 1000  600  100 ]"  Temp_C_vec="[ 45 25  ]"  ModuleName=User-defined  PlotWhenSelected=off  Pm=213.15  Ncell=60  Voc=36.3  Isc=7.84  Vm=29  Im=7.35  beta_Voc_pc=-0.36099  alpha_Isc_pc=0.102  beta_Voc=-0.13104  alpha_Isc=0.0079968  IL=7.8654  I0=2.9273e-10  nI=0.98119  Rsh=313.0553  Rs=0.39381  RobustModel=off  RobustCellTemperature=313.3991  BAL=on  Tc=1e-6  Tfilter=5e-5
  PWM Generator (DC-DC) : spsPWMGeneratorDCDCLib/PWM Generator (DC-DC)  Fsw=15e3  Ts=0
  Scope : Scope
  Series RLC Branch : spsSeriesRLCBranchLib/Series RLC Branch  LConnTagsString=__new0  RConnTagsString=__new0  BranchType=C  Resistance=0.1  Inductance=1e-3  SetiL0=off  InitialCurrent=0  Capacitance=1e-4  Setx0=on  InitialVoltage=400  Measurements=None
  Series RLC Branch1 : spsSeriesRLCBranchLib/Series RLC Branch  LConnTagsString=__new0  RConnTagsString=__new0  BranchType=L  Resistance=1  Inductance=0.1  SetiL0=off  InitialCurrent=0  Capacitance=1e-3  Setx0=off  InitialVoltage=0  Measurements=None
  Series RLC Branch3 : spsSeriesRLCBranchLib/Series RLC Branch  LConnTagsString=__new0  RConnTagsString=__new0  BranchType=RC  Resistance=0.1  Inductance=1e-3  SetiL0=off  InitialCurrent=0  Capacitance=1e-2  Setx0=on  InitialVoltage=800  Measurements=None
  Sum : Sum  Inputs=|++
  功率 : Product
  电压 : spsVoltageMeasurementLib/Voltage Measurement  PhasorSimulation=off  OutputType=Complex  PSBequivalent=0
  电压、功率 : Scope  NumInputPorts=2
  电导增量法MPPT : Subsystem
  电流 : Scope
  PV+ : PMIOPort  Side=Right
  PV- : PMIOPort  Port=2  Side=Right
  Out1 : Outport
  wires:
  Constant/1 -> "PV Array "/2  "温度"
  Sum/1 -> Scope/1, "PV Array "/1  "光照"
  Bus Selector/1 -> 电导增量法MPPT/1(V)  "<V_PV>"
  功率/1 -> [P_PV], 电压、功率/2
  Current Measurement/1 -> 功率/2, 电流/1
  电压/1 -> 功率/1, 电压、功率/1
  Bus Selector/2 -> 电导增量法MPPT/2(I)  "<I_PV>"
  "PV Array "/1 -> Bus Selector/1
  PWM Generator (DC-DC)/1 -> IGBT/1
  电导增量法MPPT/1(D) -> PWM Generator (DC-DC)/1
  [P_PV] -> Out1/1
  PV_change/1 -> Sum/2  "光照"
  Constant1/1 -> Sum/1
  connections:
  "PV Array "/RConn1 -- Series RLC Branch/LConn1 -- Current Measurement/LConn1 -- 电压/LConn1
  Series RLC Branch1/LConn1 -- IGBT/LConn1 -- Diode/LConn1
  PV-/RConn1 -- Series RLC Branch3/RConn1 -- "PV Array "/RConn2 -- 电压/LConn2 -- Series RLC Branch/RConn1 -- IGBT/RConn1
  Series RLC Branch3/LConn1 -- Diode/RConn1 -- PV+/RConn1
  Current Measurement/RConn1 -- Series RLC Branch1/RConn1

== system Microgrid_PV_WG_Bat_EV_j_22b/电解槽1 ==
  PEL_ref : Inport
  Add : Sum  Inputs=+-
  Current Measurement : spsCurrentMeasurementLib/Current Measurement  PhasorSimulation=off  OutputType=Complex  PSBequivalent=0
  Diode : spsDiodeLib/Diode  Ron=0.001  Lon=0  Vf=0.8  IC=0  UseSnubber=0  Rs=500  Cs=250e-9  Measurements=on
  Divide : Product  Inputs=*/
  IGBT/Diode : spsIGBTDiodeLib/IGBT//Diode  Ron=1e-3  Rs=1e5  Cs=inf  Measurements=on
  PID Controller1 : slpidlib/PID Controller  Controller=PI  Form=Parallel  TimeDomain=Continuous-time  UseExternalTs=off  SampleTime=-1  IntegratorMethod=Forward Euler  FilterMethod=Forward Euler  ControllerParametersSource=internal  P=100  I=5  UseKiTs=off  D=0  N=100  UseFilter=on  TunerSelectOption=Transfer Function Based (PID Tuner App)  InitialConditionSource=internal  InitialConditionForIntegrator=0  InitialConditionForFilter=0  DifferentiatorICPrevScaledInput=0  ExternalReset=none  TrackingMode=off  Kt=1  LimitOutput=off  SatLimitsSource=internal  UpperSaturationLimit=inf  LowerSaturationLimit=-inf  LinearizeAsGain=on  AntiWindupMode=none  Kb=1  LimitIntegrator=off  UpperIntegratorSaturationLimit=inf  LowerIntegratorSaturationLimit=-inf  POutMin=[]  POutMax=[]  IOutMin=[]  IOutMax=[]  DOutMin=[]  DOutMax=[]  NOutMin=[]  NOutMax=[]  SumOutMin=[]  SumOutMax=[]  SaturationOutMin=[]  SaturationOutMax=[]  PParamMin=[]  PParamMax=[]  IParamMin=[]  IParamMax=[]  DParamMin=[]  DParamMax=[]  NParamMin=[]  NParamMax=[]  KbParamMin=[]  KbParamMax=[]  KtParamMin=[]  KtParamMax=[]  KbOutMin=[]  KbOutMax=[]  KtOutMin=[]  KtOutMax=[]  IntegratorOutMin=[]  IntegratorOutMax=[]  FilterOutMin=[]  FilterOutMax=[]  SumI1OutMin=[]  SumI1OutMax=[]  SumI2OutMin=[]  SumI2OutMax=[]  SumI3OutMin=[]  SumI3OutMax=[]  SumI4OutMin=[]  SumI4OutMax=[]  SumDOutMin=[]  SumDOutMax=[]  DifferentiatorOutMin=[]  DifferentiatorOutMax=[]  FilterDiffOutCoefMin=[]  FilterDiffOutCoefMax=[]  ReciprocalOutMin=[]  ReciprocalOutMax=[]  SumDenOutMin=[]  SumDenOutMax=[]  SumNumOutMin=[]  SumNumOutMax=[]  DivideOutMin=[]  DivideOutMax=[]  UdiffTsProdOutMin=[]  UdiffTsProdOutMax=[]  NTsProdOutMin=[]  NTsProdOutMax=[]  UintegralTsProdOutMin=[]  UintegralTsProdOutMax=[]  UngainTsProdOutMin=[]  UngainTsProdOutMax=[]  IntegratorContinuousStateAttributes=''  IntegratorStateMustResolveToSignalObject=off  IntegratorRTWStateStorageClass=Auto  FilterContinuousStateAttributes=''  FilterStateMustResolveToSignalObject=off  FilterRTWStateStorageClass=Auto  ParallelPVariant=InternalParameters  IdealPVariant=Disabled  IVariant=InternalParameters  DVariant=Disabled  IntegratorVariant=Continuous  SatVariant=Disabled  AWVariant=Passthrough  PCopyVariant=Disabled  TRVariant=Disabled  FdbkBlocksVariant=Forward  IdealPFdbkVariant=Disabled  SatFdbkVariant=Disabled  DerivativeFilterVariant=Disabled  NVariant=Disabled  NCopyVariant=Disabled_SignalSpec  FilterICVariant=Disabled  IntegratorICVariant=InternalICs  ExternalResetVariant=Disabled  TRSumVariant=Passthrough  SumFdbkVariant=Disabled  SumVariant=Sum_PI  TsampFilterVariant=InternalTs  TsampNgainVariant=Passthrough  TsampIntegralVariant=Disabled_SignalSpec  ExternalSaturationOutDataTypeStr=Inherit: Same as second input
  PWM Generator (DC-DC) : spsPWMGeneratorDCDCLib/PWM Generator (DC-DC)  Fsw=1e4  Ts=0
  Product : Product
  Scope : Scope
  Scope1 : Scope
  Scope2 : Scope
  Series RLC Branch : spsSeriesRLCBranchLib/Series RLC Branch  LConnTagsString=__new0  RConnTagsString=__new0  BranchType=L  Resistance=1  Inductance=5e-2  SetiL0=off  InitialCurrent=0  Capacitance=1e-6  Setx0=off  InitialVoltage=0  Measurements=None
  Voltage Measurement1 : spsVoltageMeasurementLib/Voltage Measurement  PhasorSimulation=off  OutputType=Complex  PSBequivalent=0
  Zero-Order Hold : ZeroOrderHold  SampleTime=1e-5
  Zero-Order Hold3 : ZeroOrderHold  SampleTime=1e-5
  功率参考值 : Constant  Value=12e5
  电解池 : Subsystem
  EL+ : PMIOPort  Side=Left
  EL- : PMIOPort  Port=2  Side=Left
  Velec mol/s : Outport
  Uelec : Outport  Port=2
  Ielec : Outport  Port=3
  wires:
  [I] -> Product/1, Scope/1
  Product/1 -> Scope2/1
  Zero-Order Hold3/1 -> Divide/2
  Voltage Measurement1/1 -> [V]
  [PWM] -> IGBT/Diode/1
  [V] -> Uelec/1, Zero-Order Hold3/1
  Zero-Order Hold/1 -> Add/2
  [I] -> Ielec/1, Zero-Order Hold/1
  PEL_ref/1 -> Divide/1
  PWM Generator (DC-DC)/1 -> [PWM]
  Add/1 -> PID Controller1/1
  Divide/1 -> Add/1
  PID Controller1/1 -> PWM Generator (DC-DC)/1
  Current Measurement/1 -> [I]
  [V] -> Product/2, Scope1/1
  电解池/1(产氢速率 mol/s) -> Velec mol/s/1
  connections:
  Diode/LConn1 -- EL-/RConn1 -- 电解池/LConn2 -- Voltage Measurement1/LConn2
  Current Measurement/LConn1 -- Series RLC Branch/RConn1
  EL+/RConn1 -- IGBT/Diode/LConn1
  Current Measurement/RConn1 -- Voltage Measurement1/LConn1 -- 电解池/LConn1
  Diode/RConn1 -- Series RLC Branch/LConn1 -- IGBT/Diode/RConn1

== system Microgrid_PV_WG_Bat_EV_j_22b/逆变器整流 ==
  Current Measurement : spsCurrentMeasurementLib/Current Measurement  PhasorSimulation=off  OutputType=Complex  PSBequivalent=0
  Scope13 : Scope
  Scope20 : Scope
  Series RLC Branch1 : spsSeriesRLCBranchLib/Series RLC Branch  LConnTagsString=__new0  RConnTagsString=__new0  BranchType=RC  Resistance=0.05  Inductance=1e-3  SetiL0=off  InitialCurrent=0  Capacitance=8e-3  Setx0=on  InitialVoltage=1800  Measurements=None
  Three-Phase Series RLC Branch3 : spsThreePhaseSeriesRLCBranchLib/Three-Phase Series RLC Branch  LConnTagsString=A|B|C  RConnTagsString=A|B|C  BranchType=RL  Resistance=0.05  Inductance=7e-3  Capacitance=1e-6  Measurements=None
  Three-Phase V-I Measurement4 : spsThreePhaseVIMeasurementLib/Three-Phase V-I Measurement  VoltageMeasurement=phase-to-ground  SetLabelV=on  LabelV=Vabc_EV  Vpu=off  VpuLL=off  CurrentMeasurement=yes  SetLabelI=on  LabelI=Iabc_EV  Ipu=off  Pbase=100e6  Vbase=500e3  OutputType=Complex  PhasorSimulation=off  PSBequivalent=0
  Universal Bridge2 : spsUniversalBridgeLib/Universal Bridge  Arms=3  SnubberResistance=1e5  SnubberCapacitance=inf  Device=IGBT / Diodes  Ron=1e-3  Lon=0  ForwardVoltages="[  0  0  ]"  ForwardVoltage=0  GTOparameters=[ 10e-6 , 20e-6 ]  IGBTparameters=[ 1e-6 , 2e-6 ]  Measurements=None  Measurements_2=None  converterType=Rectifier
  Uref : Constant  Value=1000
  Voltage Measurement2 : spsVoltageMeasurementLib/Voltage Measurement  PhasorSimulation=off  OutputType=Complex  PSBequivalent=0
  controller2 : Subsystem
  + : PMIOPort  Side=Left
  a : PMIOPort  Port=2  Side=Right
  b : PMIOPort  Port=3  Side=Right
  - : PMIOPort  Port=4  Side=Left
  c : PMIOPort  Port=5  Side=Right
  wires:
  [Iabc_EV] -> controller2/4(Iabc)
  [PWM] -> Universal Bridge2/1
  Current Measurement/1 -> Scope20/1
  Voltage Measurement2/1 -> [Vdc], Scope13/1
  [Vabc_EV] -> controller2/3(Vabc)
  [Vdc] -> controller2/1(Udc)
  controller2/1(Pulse) -> [PWM]
  Uref/1 -> controller2/2(Udc_ref)
  connections:
  Universal Bridge2/LConn1 -- Three-Phase Series RLC Branch3/LConn1
  Three-Phase Series RLC Branch3/RConn1 -- Three-Phase V-I Measurement4/LConn1
  Current Measurement/RConn1 -- +/RConn1 -- Series RLC Branch1/LConn1
  Universal Bridge2/RConn2 -- -/RConn1 -- Series RLC Branch1/RConn1 -- Voltage Measurement2/LConn2
  Three-Phase Series RLC Branch3/LConn3 -- Universal Bridge2/LConn3
  Three-Phase Series RLC Branch3/LConn2 -- Universal Bridge2/LConn2
  Universal Bridge2/RConn1 -- Current Measurement/LConn1 -- Voltage Measurement2/LConn1
  Three-Phase Series RLC Branch3/RConn3 -- Three-Phase V-I Measurement4/LConn3
  Three-Phase Series RLC Branch3/RConn2 -- Three-Phase V-I Measurement4/LConn2
  a/RConn1 -- Three-Phase V-I Measurement4/RConn1
  b/RConn1 -- Three-Phase V-I Measurement4/RConn2
  c/RConn1 -- Three-Phase V-I Measurement4/RConn3

== system Microgrid_PV_WG_Bat_EV_j_22b/逆变器整流1 ==
  Current Measurement : spsCurrentMeasurementLib/Current Measurement  PhasorSimulation=off  OutputType=Complex  PSBequivalent=0
  Scope13 : Scope
  Scope20 : Scope
  Series RLC Branch1 : spsSeriesRLCBranchLib/Series RLC Branch  LConnTagsString=__new0  RConnTagsString=__new0  BranchType=RC  Resistance=0.05  Inductance=1e-3  SetiL0=off  InitialCurrent=0  Capacitance=8e-3  Setx0=on  InitialVoltage=800  Measurements=None
  Three-Phase Series RLC Branch3 : spsThreePhaseSeriesRLCBranchLib/Three-Phase Series RLC Branch  LConnTagsString=A|B|C  RConnTagsString=A|B|C  BranchType=RL  Resistance=0.05  Inductance=7e-3  Capacitance=1e-6  Measurements=None
  Three-Phase V-I Measurement4 : spsThreePhaseVIMeasurementLib/Three-Phase V-I Measurement  VoltageMeasurement=phase-to-ground  SetLabelV=on  LabelV=Vabc_PEL  Vpu=off  VpuLL=off  CurrentMeasurement=yes  SetLabelI=on  LabelI=Iabc_PEL  Ipu=off  Pbase=100e6  Vbase=500e3  OutputType=Complex  PhasorSimulation=off  PSBequivalent=0
  Universal Bridge2 : spsUniversalBridgeLib/Universal Bridge  Arms=3  SnubberResistance=1e5  SnubberCapacitance=inf  Device=IGBT / Diodes  Ron=1e-3  Lon=0  ForwardVoltages="[  0  0  ]"  ForwardVoltage=0  GTOparameters=[ 10e-6 , 20e-6 ]  IGBTparameters=[ 1e-6 , 2e-6 ]  Measurements=None  Measurements_2=None  converterType=Rectifier
  Uref : Constant  Value=1000
  Voltage Measurement2 : spsVoltageMeasurementLib/Voltage Measurement  PhasorSimulation=off  OutputType=Complex  PSBequivalent=0
  controller2 : Subsystem
  + : PMIOPort  Side=Left
  a : PMIOPort  Port=2  Side=Right
  b : PMIOPort  Port=3  Side=Right
  - : PMIOPort  Port=4  Side=Left
  c : PMIOPort  Port=5  Side=Right
  wires:
  [Iabc_PEL] -> controller2/4(Iabc)
  [PWM] -> Universal Bridge2/1
  Current Measurement/1 -> Scope20/1
  Voltage Measurement2/1 -> [Vdc], Scope13/1
  [Vabc_PEL] -> controller2/3(Vabc)
  [Vdc] -> controller2/1(Udc)
  controller2/1(Pulse) -> [PWM]
  Uref/1 -> controller2/2(Udc_ref)
  connections:
  Universal Bridge2/LConn1 -- Three-Phase Series RLC Branch3/LConn1
  Three-Phase Series RLC Branch3/RConn1 -- Three-Phase V-I Measurement4/LConn1
  Current Measurement/RConn1 -- +/RConn1 -- Series RLC Branch1/LConn1
  Series RLC Branch1/RConn1 -- -/RConn1 -- Universal Bridge2/RConn2 -- Voltage Measurement2/LConn2
  Three-Phase Series RLC Branch3/LConn3 -- Universal Bridge2/LConn3
  Three-Phase Series RLC Branch3/LConn2 -- Universal Bridge2/LConn2
  Universal Bridge2/RConn1 -- Voltage Measurement2/LConn1 -- Current Measurement/LConn1
  Three-Phase Series RLC Branch3/RConn3 -- Three-Phase V-I Measurement4/LConn3
  Three-Phase Series RLC Branch3/RConn2 -- Three-Phase V-I Measurement4/LConn2
  a/RConn1 -- Three-Phase V-I Measurement4/RConn1
  b/RConn1 -- Three-Phase V-I Measurement4/RConn2
  c/RConn1 -- Three-Phase V-I Measurement4/RConn3

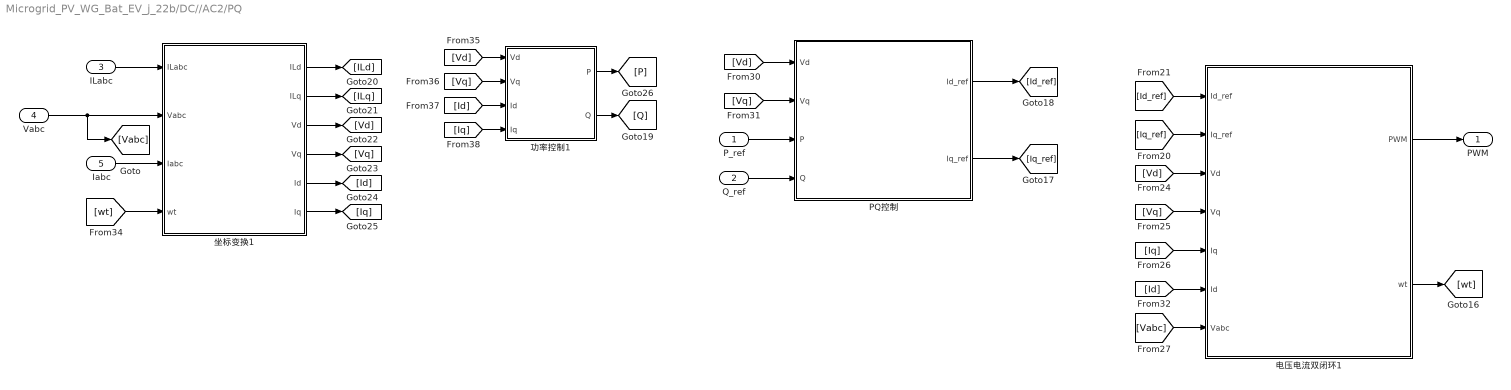
== system Microgrid_PV_WG_Bat_EV_j_22b/DC//AC2/PQ ==
  P_ref : Inport
  Q_ref : Inport  Port=2
  ILabc : Inport  Port=3
  Vabc : Inport  Port=4
  Iabc : Inport  Port=5
  PQ控制 : Subsystem
  功率控制1 : Subsystem
  坐标变换1 : Subsystem
  电压电流双闭环1 : Subsystem
  PWM : Outport
  wires:
  坐标变换1/6(Iq) -> [Iq]
  [Id_ref] -> 电压电流双闭环1/1(Id_ref)
  功率控制1/1(P) -> [P]
  P_ref/1 -> PQ控制/3(P)
  电压电流双闭环1/1(PWM) -> PWM/1
  坐标变换1/4(Vq) -> [Vq]
  PQ控制/2(Iq_ref) -> [Iq_ref]
  [Vq] -> PQ控制/2(Vq)
  [Vabc] -> 电压电流双闭环1/7(Vabc)
  坐标变换1/5(Id) -> [Id]
  [Vq] -> 电压电流双闭环1/4(Vq)
  [wt] -> 坐标变换1/4(wt)
  [Vd] -> 电压电流双闭环1/3(Vd)
  [Iq] -> 电压电流双闭环1/5(Iq)
  [Id] -> 电压电流双闭环1/6(Id)
  [Vq] -> 功率控制1/2(Vq)
  [Vd] -> PQ控制/1(Vd)
  坐标变换1/1(ILd) -> [ILd]
  Q_ref/1 -> PQ控制/4(Q)
  PQ控制/1(Id_ref) -> [Id_ref]
  电压电流双闭环1/2(wt) -> [wt]
  [Vd] -> 功率控制1/1(Vd)
  [Iq_ref] -> 电压电流双闭环1/2(Iq_ref)
  ILabc/1 -> 坐标变换1/1(ILabc)
  坐标变换1/3(Vd) -> [Vd]
  坐标变换1/2(ILq) -> [ILq]
  [Id] -> 功率控制1/3(Id)
  [Iq] -> 功率控制1/4(Iq)
  功率控制1/2(Q) -> [Q]
  Iabc/1 -> 坐标变换1/3(Iabc)
  Vabc/1 -> 坐标变换1/2(Vabc), [Vabc]

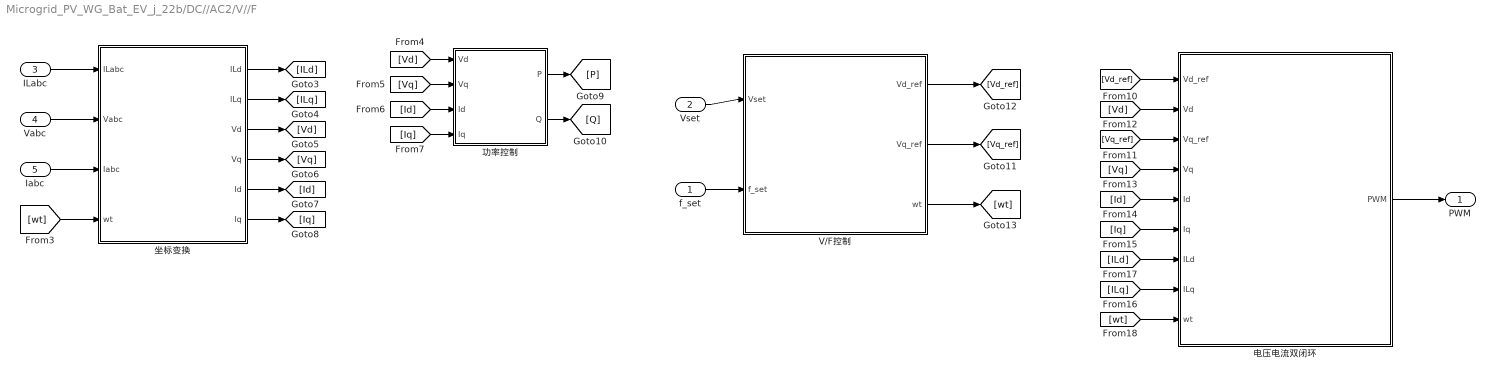
== system Microgrid_PV_WG_Bat_EV_j_22b/DC//AC2/V//F ==
  f_set : Inport
  Vset : Inport  Port=2
  ILabc : Inport  Port=3
  Vabc : Inport  Port=4
  Iabc : Inport  Port=5
  V/F控制 : Subsystem
  功率控制 : Subsystem
  坐标变换 : Subsystem
  电压电流双闭环 : Subsystem
  PWM : Outport
  wires:
  坐标变换/3(Vd) -> [Vd]
  Vset/1 -> V/F控制/1(Vset)
  [Vd_ref] -> 电压电流双闭环/1(Vd_ref)
  ILabc/1 -> 坐标变换/1(ILabc)
  功率控制/2(Q) -> [Q]
  Iabc/1 -> 坐标变换/3(Iabc)
  坐标变换/4(Vq) -> [Vq]
  [wt] -> 电压电流双闭环/9(wt)
  V/F控制/2(Vq_ref) -> [Vq_ref]
  V/F控制/3(wt) -> [wt]
  Vabc/1 -> 坐标变换/2(Vabc)
  [Vd] -> 功率控制/1(Vd)
  [ILq] -> 电压电流双闭环/8(ILq)
  [wt] -> 坐标变换/4(wt)
  [Iq] -> 电压电流双闭环/6(Iq)
  [ILd] -> 电压电流双闭环/7(ILd)
  V/F控制/1(Vd_ref) -> [Vd_ref]
  [Vq] -> 功率控制/2(Vq)
  坐标变换/6(Iq) -> [Iq]
  [Vq] -> 电压电流双闭环/4(Vq)
  [Id] -> 功率控制/3(Id)
  功率控制/1(P) -> [P]
  坐标变换/2(ILq) -> [ILq]
  [Vd] -> 电压电流双闭环/2(Vd)
  [Iq] -> 功率控制/4(Iq)
  坐标变换/5(Id) -> [Id]
  电压电流双闭环/1(PWM) -> PWM/1
  [Id] -> 电压电流双闭环/5(Id)
  [Vq_ref] -> 电压电流双闭环/3(Vq_ref)
  坐标变换/1(ILd) -> [ILd]
  f_set/1 -> V/F控制/2(f_set)

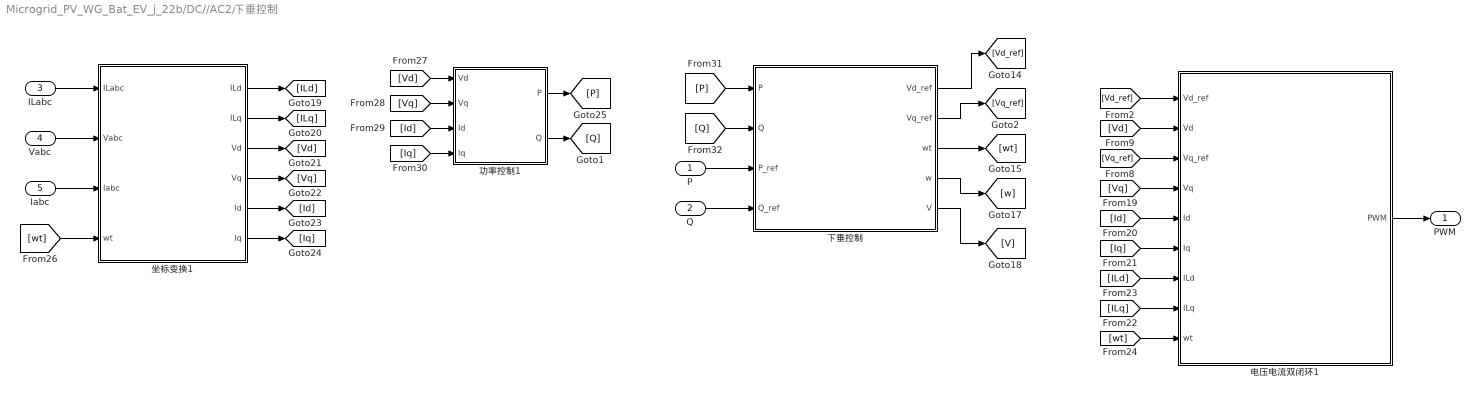
== system Microgrid_PV_WG_Bat_EV_j_22b/DC//AC2/下垂控制 ==
  P : Inport
  Q : Inport  Port=2
  ILabc : Inport  Port=3
  Vabc : Inport  Port=4
  Iabc : Inport  Port=5
  下垂控制 : Subsystem
  功率控制1 : Subsystem
  坐标变换1 : Subsystem
  电压电流双闭环1 : Subsystem
  PWM : Outport
  wires:
  [Vq] -> 电压电流双闭环1/4(Vq)
  坐标变换1/2(ILq) -> [ILq]
  [Q] -> 下垂控制/2(Q)
  坐标变换1/3(Vd) -> [Vd]
  [Vq_ref] -> 电压电流双闭环1/3(Vq_ref)
  坐标变换1/1(ILd) -> [ILd]
  Vabc/1 -> 坐标变换1/2(Vabc)
  ILabc/1 -> 坐标变换1/1(ILabc)
  [wt] -> 电压电流双闭环1/9(wt)
  坐标变换1/5(Id) -> [Id]
  坐标变换1/6(Iq) -> [Iq]
  [Vq] -> 功率控制1/2(Vq)
  [Iq] -> 功率控制1/4(Iq)
  Iabc/1 -> 坐标变换1/3(Iabc)
  [wt] -> 坐标变换1/4(wt)
  坐标变换1/4(Vq) -> [Vq]
  [Iq] -> 电压电流双闭环1/6(Iq)
  下垂控制/5(V) -> [V]
  下垂控制/3(wt) -> [wt]
  [Vd_ref] -> 电压电流双闭环1/1(Vd_ref)
  下垂控制/2(Vq_ref) -> [Vq_ref]
  Q/1 -> 下垂控制/4(Q_ref)
  [Id] -> 功率控制1/3(Id)
  [Id] -> 电压电流双闭环1/5(Id)
  电压电流双闭环1/1(PWM) -> PWM/1
  [P] -> 下垂控制/1(P)
  功率控制1/2(Q) -> [Q]
  下垂控制/4(w) -> [w]
  [ILd] -> 电压电流双闭环1/7(ILd)
  P/1 -> 下垂控制/3(P_ref)
  [Vd] -> 功率控制1/1(Vd)
  功率控制1/1(P) -> [P]
  [Vd] -> 电压电流双闭环1/2(Vd)
  下垂控制/1(Vd_ref) -> [Vd_ref]
  [ILq] -> 电压电流双闭环1/8(ILq)

== system Microgrid_PV_WG_Bat_EV_j_22b/Subsystem/电压外环控制，控制直流母线电压为目标值 ==
  In1 : Inport
  In2 : Inport  Port=2
  PID Controller2 : slpidlib/PID Controller  Controller=PID  Form=Parallel  TimeDomain=Continuous-time  UseExternalTs=off  SampleTime=-1  IntegratorMethod=Forward Euler  FilterMethod=Forward Euler  ControllerParametersSource=internal  P=1  I=10  UseKiTs=off  D=0  N=100  UseFilter=on  TunerSelectOption=Transfer Function Based (PID Tuner App)  InitialConditionSource=internal  InitialConditionForIntegrator=0  InitialConditionForFilter=0  DifferentiatorICPrevScaledInput=0  ExternalReset=none  TrackingMode=off  Kt=1  LimitOutput=off  SatLimitsSource=internal  UpperSaturationLimit=inf  LowerSaturationLimit=-inf  LinearizeAsGain=on  AntiWindupMode=none  Kb=1  LimitIntegrator=off  UpperIntegratorSaturationLimit=inf  LowerIntegratorSaturationLimit=-inf  POutMin=[]  POutMax=[]  IOutMin=[]  IOutMax=[]  DOutMin=[]  DOutMax=[]  NOutMin=[]  NOutMax=[]  SumOutMin=[]  SumOutMax=[]  SaturationOutMin=[]  SaturationOutMax=[]  PParamMin=[]  PParamMax=[]  IParamMin=[]  IParamMax=[]  DParamMin=[]  DParamMax=[]  NParamMin=[]  NParamMax=[]  KbParamMin=[]  KbParamMax=[]  KtParamMin=[]  KtParamMax=[]  KbOutMin=[]  KbOutMax=[]  KtOutMin=[]  KtOutMax=[]  IntegratorOutMin=[]  IntegratorOutMax=[]  FilterOutMin=[]  FilterOutMax=[]  SumI1OutMin=[]  SumI1OutMax=[]  SumI2OutMin=[]  SumI2OutMax=[]  SumI3OutMin=[]  SumI3OutMax=[]  SumI4OutMin=[]  SumI4OutMax=[]  SumDOutMin=[]  SumDOutMax=[]  DifferentiatorOutMin=[]  DifferentiatorOutMax=[]  FilterDiffOutCoefMin=[]  FilterDiffOutCoefMax=[]  ReciprocalOutMin=[]  ReciprocalOutMax=[]  SumDenOutMin=[]  SumDenOutMax=[]  SumNumOutMin=[]  SumNumOutMax=[]  DivideOutMin=[]  DivideOutMax=[]  UdiffTsProdOutMin=[]  UdiffTsProdOutMax=[]  NTsProdOutMin=[]  NTsProdOutMax=[]  UintegralTsProdOutMin=[]  UintegralTsProdOutMax=[]  UngainTsProdOutMin=[]  UngainTsProdOutMax=[]  IntegratorContinuousStateAttributes=''  IntegratorStateMustResolveToSignalObject=off  IntegratorRTWStateStorageClass=Auto  FilterContinuousStateAttributes=''  FilterStateMustResolveToSignalObject=off  FilterRTWStateStorageClass=Auto  ParallelPVariant=InternalParameters  IdealPVariant=Disabled  IVariant=InternalParameters  DVariant=InternalParameters  IntegratorVariant=Continuous  SatVariant=Disabled  AWVariant=Passthrough  PCopyVariant=Disabled  TRVariant=Disabled  FdbkBlocksVariant=Forward  IdealPFdbkVariant=Disabled  SatFdbkVariant=Disabled  DerivativeFilterVariant=ContFilter  NVariant=InternalParameters  NCopyVariant=Disabled  FilterICVariant=InternalICsFilter  IntegratorICVariant=InternalICs  ExternalResetVariant=Disabled  TRSumVariant=Passthrough  SumFdbkVariant=Disabled  SumVariant=Sum_PID  TsampFilterVariant=InternalTs  TsampNgainVariant=Passthrough  TsampIntegralVariant=Disabled_SignalSpec  ExternalSaturationOutDataTypeStr=Inherit: Same as second input
  Saturation : Saturate  UpperLimit=100  LowerLimit=1
  Subtract : Sum  Inputs=+-
  Out1 : Outport
  wires:
  Subtract/1 -> PID Controller2/1
  PID Controller2/1 -> Saturation/1
  In1/1 -> Subtract/1
  In2/1 -> Subtract/2
  Saturation/1 -> Out1/1
